simulink model "Sfun_dtc_ASR"  (Simulink 8.5)
settings: Solver=ode3  StartTime=0.0  StopTime=1  FixedStep=1e-5  RelTol=1e-3  AbsTol=1e-5
PreLoadFcn:
  | Ts=1e-5;
  | load srm64_60kw
undefined symbols (not defined in the file or in its folder): find_system
libraries: powerlib x15, simulink x1
Description:
  | Copyright 2008-2010 The MathWorks, Inc.
settings Model: Creator=MathWorks  LastModifiedBy=think0404  ExtModeAutoUpdateStatusClock=off
settings DataIOCC: SignalLoggingName=sigsOut
settings OptimizationCC: InitFltsAndDblsToZero=on
settings DebuggingCC: CheckExecutionContextPreStartOutputMsg=on  CheckExecutionContextRuntimeOutputMsg=on  SignalResolutionControl=TryResolveAllWithWarning  MultiTaskDSMMsg=warning  MultiTaskCondExecSysMsg=none  FcnCallInpInsideContextMsg=UseLocalSettings
settings HardwareCC: TargetUnknown=on

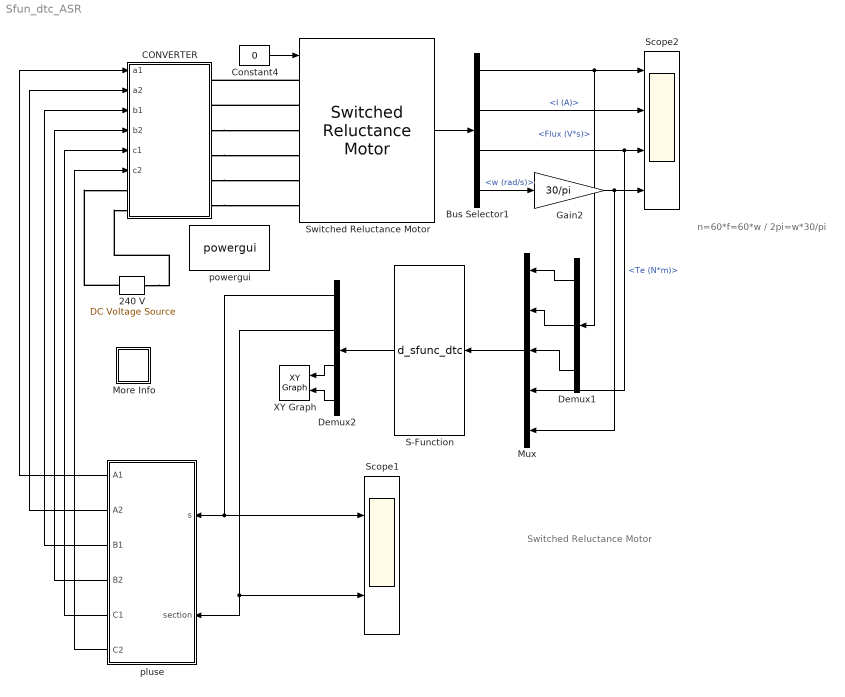
== system Sfun_dtc_ASR ==
  note: Switched Reluctance Motor
  note: n=60*f=60*w / 2pi=w*30/pi
  240 V : powerlib/Electrical Sources/DC Voltage Source  Amplitude=300  Measurements=None
  Bus Selector1 : BusSelector  OutputSignals=Flux (V*s),I (A),Te (N*m),w (rad/s)
  CONVERTER : Subsystem  LoadFcn=find_system(gcs,'FollowLinks', 'on', 'LookUnderMasks', 'all');
  Constant4 : Constant  Value=0
  Demux1 : Demux  Outputs=3
  Demux2 : Demux
  Gain2 : Gain  Gain=30/pi  SaturateOnIntegerOverflow=on  OutDataTypeStr=Inherit: Same as input  ParamDataTypeStr=Inherit: Same as input
  More Info : Subsystem
      settings: OpenFcn=showdemo(bdroot(gcb))
      mask Display: disp('?')
  Mux : Mux  Inputs=5
  S-Function : S-Function  FunctionName=d_sfunc_dtc  Parameters=0.25,3000,1e-4,1e-3,30
  Scope1 : Scope  NumInputPorts=2
      settings: TimeRange=0.1  YMin=1~1  YMax=4~6  SaveName=VI1  Decimation=10
  Scope2 : Scope  NumInputPorts=4
      settings: TimeRange=1  YMin=-0.05~-50~-200~-500  YMax=0.35~550~150~4500  SaveName=VI  Decimation=10
  Switched Reluctance Motor : powerlib/Machines/Switched Reluctance Motor  MachineType=6/4  StatorResistance=0.05  Inertia=0.05  Friction=0.02  InitialSpeed=[0,0]  TsPowergui=0  TsBlock=-1  MachineModel=Generic model  Lq=0.67e-3  Ld=23.6e-3  Lsat=0.15e-3  MaximumCurrent=450  MaximumFluxLinkage=0.486  Source=MAT-file  MagnetisationCharacteristic='srm64_60kw.mat'  RotorAngleVector=[0 10 20 30 40 45]  StatorCurrentVector=0:25:450  PlotCurves=off
  XY Graph : simulink/Sinks/XY Graph  xmin=-1  xmax=1  ymin=-1  ymax=1  st=-1
  pluse : Subsystem
  powergui : powerlib/powergui  Priority=2  SimulationMode=Discrete  SolverType=Tustin/Backward Euler (TBE)  SampleTime=1e-5  frequency=60  SPID=off  DisableSnubberDevices=off  DisableRonSwitches=off  DisableVfSwitches=off  SwTol=0  DisplayEquations=off  Interpol=off  methode=off  Ts=0  FunctionMessages=off  echomessages=off  HookPort=off  EnableUseOfTLC=off  x0status=blocks  frequencyindice=0  Pbase=100e6  ErrMax=1e-4  Iterations=50  UnitsV=kV  UnitsW=MW  buscounter=0  RestoreLinks=warning  ResistiveCurrentMeasurement=off  Frange=[0:2:500]  Ylog=off  Xlog=on  ShowGrid=off  save=off  variable=ZData  structure=0  ZoomFFT=on  StartTime=0.0  cycles=1  DisplayStyle=1  fundamental=60  FreqAxis=off  MaxFrequency=1000  frequencyindicesteady=1  RmsSteady=1  display=off
  wires:
  Constant4/1 -> Switched Reluctance Motor/1
  Switched Reluctance Motor/1 -> Bus Selector1/1
  Bus Selector1/1 -> Scope2/1, Demux1/1  "<Flux (V*s)>"
  Bus Selector1/2 -> Scope2/2  "<I (A)>"
  Bus Selector1/3 -> Scope2/3, Mux/4  "<Te (N*m)>"
  Gain2/1 -> Scope2/4, Mux/5
  Bus Selector1/4 -> Gain2/1  "<w (rad/s)>"
  pluse/1(A1) -> CONVERTER/1(a1)
  pluse/2(A2) -> CONVERTER/2(a2)
  pluse/3(B1) -> CONVERTER/3(b1)
  pluse/4(B2) -> CONVERTER/4(b2)
  pluse/5(C1) -> CONVERTER/5(c1)
  pluse/6(C2) -> CONVERTER/6(c2)
  Demux1/1 -> Mux/1
  Demux1/2 -> Mux/2
  Demux1/3 -> Mux/3
  Mux/1 -> S-Function/1
  S-Function/1 -> Demux2/1
  Demux2/1 -> pluse/1(s), Scope1/1
  Demux2/2 -> pluse/2(section), Scope1/2
  Demux2/3 -> XY Graph/1
  Demux2/4 -> XY Graph/2
  connections:
  Switched Reluctance Motor/LConn1 -- CONVERTER/RConn1
  Switched Reluctance Motor/LConn2 -- CONVERTER/RConn2
  CONVERTER/RConn3 -- Switched Reluctance Motor/LConn3
  CONVERTER/RConn4 -- Switched Reluctance Motor/LConn4
  CONVERTER/RConn5 -- Switched Reluctance Motor/LConn5
  CONVERTER/RConn6 -- Switched Reluctance Motor/LConn6
  240 V/RConn1 -- CONVERTER/LConn1
  240 V/LConn1 -- CONVERTER/LConn2

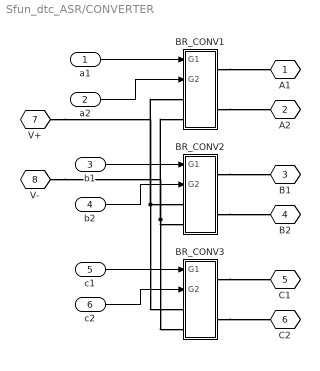
== system Sfun_dtc_ASR/CONVERTER ==
  a1 : Inport
  a2 : Inport  Port=2
  b1 : Inport  Port=3
  b2 : Inport  Port=4
  c1 : Inport  Port=5
  c2 : Inport  Port=6
  BR_CONV1 : Subsystem
  BR_CONV2 : Subsystem
  BR_CONV3 : Subsystem
  A1 : PMIOPort  Tag=PMCPort  Port=1  Side=Right
  A2 : PMIOPort  Tag=PMCPort  Port=2  Side=Right
  B1 : PMIOPort  Tag=PMCPort  Port=3  Side=Right
  B2 : PMIOPort  Tag=PMCPort  Port=4  Side=Right
  C1 : PMIOPort  Tag=PMCPort  Port=5  Side=Right
  C2 : PMIOPort  Tag=PMCPort  Port=6  Side=Right
  V+ : PMIOPort  Tag=PMCPort  Port=7  Side=Left
  V- : PMIOPort  Tag=PMCPort  Port=8  Side=Left
  wires:
  a1/1 -> BR_CONV1/1(G1)
  a2/1 -> BR_CONV1/2(G2)
  b1/1 -> BR_CONV2/1(G1)
  b2/1 -> BR_CONV2/2(G2)
  c1/1 -> BR_CONV3/1(G1)
  c2/1 -> BR_CONV3/2(G2)
  connections:
  BR_CONV3/RConn2 -- C2/RConn1
  BR_CONV3/RConn1 -- C1/RConn1
  BR_CONV2/RConn2 -- B2/RConn1
  BR_CONV2/RConn1 -- B1/RConn1
  BR_CONV1/RConn2 -- A2/RConn1
  BR_CONV1/RConn1 -- A1/RConn1
  V+/RConn1 -- BR_CONV1/LConn1 -- BR_CONV2/LConn1 -- BR_CONV3/LConn1
  V-/RConn1 -- BR_CONV1/LConn2 -- BR_CONV2/LConn2 -- BR_CONV3/LConn2

== system Sfun_dtc_ASR/More Info ==

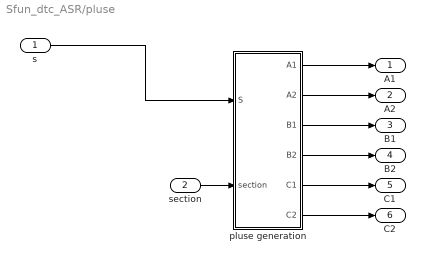
== system Sfun_dtc_ASR/pluse ==
  s : Inport
  section : Inport  Port=2
  pluse generation : Subsystem
  A1 : Outport
  A2 : Outport  Port=2
  B1 : Outport  Port=3
  B2 : Outport  Port=4
  C1 : Outport  Port=5
  C2 : Outport  Port=6
  wires:
  s/1 -> pluse generation/1(S)
  section/1 -> pluse generation/2(section)
  pluse generation/1(A1) -> A1/1
  pluse generation/2(A2) -> A2/1
  pluse generation/3(B1) -> B1/1
  pluse generation/4(B2) -> B2/1
  pluse generation/5(C1) -> C1/1
  pluse generation/6(C2) -> C2/1

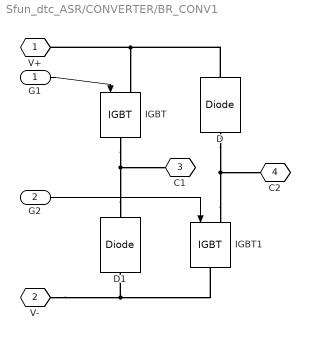
== system Sfun_dtc_ASR/CONVERTER/BR_CONV1 ==
  G1 : Inport
  G2 : Inport  Port=2
  D : powerlib/Power Electronics/Diode  Ron=1e-3  Lon=0  Vf=0.8  IC=0  UseSnubber=off  Rs=1000  Cs=inf  Measurements=off
  D1 : powerlib/Power Electronics/Diode  Ron=1e-3  Lon=0  Vf=0.8  IC=0  UseSnubber=off  Rs=1000  Cs=inf  Measurements=off
  IGBT : powerlib/Power Electronics/IGBT  Ron=1e-3  Lon=0  Vf=1  Tf=0  Tt=0  IC=0  Rs=200  Cs=0.1e-6  Measurements=off
  IGBT1 : powerlib/Power Electronics/IGBT  Ron=1e-3  Lon=0  Vf=1  Tf=0  Tt=0  IC=0  Rs=200  Cs=0.1e-6  Measurements=off
  V+ : PMIOPort  Tag=PMCPort  Port=1  Side=Left
  V- : PMIOPort  Tag=PMCPort  Port=2  Side=Left
  C1 : PMIOPort  Tag=PMCPort  Port=3  Side=Right
  C2 : PMIOPort  Tag=PMCPort  Port=4  Side=Right
  wires:
  G2/1 -> IGBT1/1
  G1/1 -> IGBT/1
  connections:
  D1/LConn1 -- V-/RConn1 -- IGBT1/RConn1
  IGBT1/LConn1 -- D/LConn1 -- C2/RConn1
  D1/RConn1 -- IGBT/RConn1 -- C1/RConn1
  D/RConn1 -- V+/RConn1 -- IGBT/LConn1

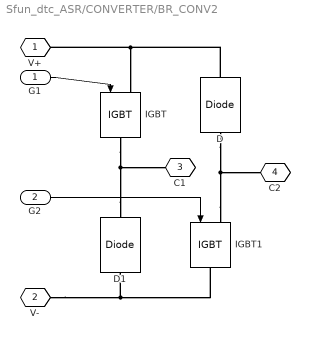
== system Sfun_dtc_ASR/CONVERTER/BR_CONV2 ==
  G1 : Inport
  G2 : Inport  Port=2
  D : powerlib/Power Electronics/Diode  Ron=1e-3  Lon=0  Vf=0.8  IC=0  UseSnubber=off  Rs=1000  Cs=inf  Measurements=off
  D1 : powerlib/Power Electronics/Diode  Ron=1e-3  Lon=0  Vf=0.8  IC=0  UseSnubber=off  Rs=1000  Cs=inf  Measurements=off
  IGBT : powerlib/Power Electronics/IGBT  Ron=1e-3  Lon=0  Vf=1  Tf=0  Tt=0  IC=0  Rs=200  Cs=0.1e-6  Measurements=off
  IGBT1 : powerlib/Power Electronics/IGBT  Ron=1e-3  Lon=0  Vf=1  Tf=0  Tt=0  IC=0  Rs=200  Cs=0.1e-6  Measurements=off
  V+ : PMIOPort  Tag=PMCPort  Port=1  Side=Left
  V- : PMIOPort  Tag=PMCPort  Port=2  Side=Left
  C1 : PMIOPort  Tag=PMCPort  Port=3  Side=Right
  C2 : PMIOPort  Tag=PMCPort  Port=4  Side=Right
  wires:
  G2/1 -> IGBT1/1
  G1/1 -> IGBT/1
  connections:
  D1/LConn1 -- V-/RConn1 -- IGBT1/RConn1
  IGBT1/LConn1 -- D/LConn1 -- C2/RConn1
  D1/RConn1 -- IGBT/RConn1 -- C1/RConn1
  D/RConn1 -- V+/RConn1 -- IGBT/LConn1

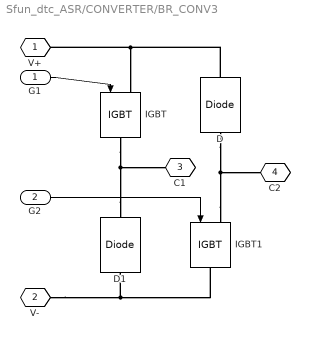
== system Sfun_dtc_ASR/CONVERTER/BR_CONV3 ==
  G1 : Inport
  G2 : Inport  Port=2
  D : powerlib/Power Electronics/Diode  Ron=1e-3  Lon=0  Vf=0.8  IC=0  UseSnubber=off  Rs=1000  Cs=inf  Measurements=off
  D1 : powerlib/Power Electronics/Diode  Ron=1e-3  Lon=0  Vf=0.8  IC=0  UseSnubber=off  Rs=1000  Cs=inf  Measurements=off
  IGBT : powerlib/Power Electronics/IGBT  Ron=1e-3  Lon=0  Vf=1  Tf=0  Tt=0  IC=0  Rs=200  Cs=0.1e-6  Measurements=off
  IGBT1 : powerlib/Power Electronics/IGBT  Ron=1e-3  Lon=0  Vf=1  Tf=0  Tt=0  IC=0  Rs=200  Cs=0.1e-6  Measurements=off
  V+ : PMIOPort  Tag=PMCPort  Port=1  Side=Left
  V- : PMIOPort  Tag=PMCPort  Port=2  Side=Left
  C1 : PMIOPort  Tag=PMCPort  Port=3  Side=Right
  C2 : PMIOPort  Tag=PMCPort  Port=4  Side=Right
  wires:
  G2/1 -> IGBT1/1
  G1/1 -> IGBT/1
  connections:
  D1/LConn1 -- V-/RConn1 -- IGBT1/RConn1
  IGBT1/LConn1 -- D/LConn1 -- C2/RConn1
  D1/RConn1 -- IGBT/RConn1 -- C1/RConn1
  D/RConn1 -- V+/RConn1 -- IGBT/LConn1

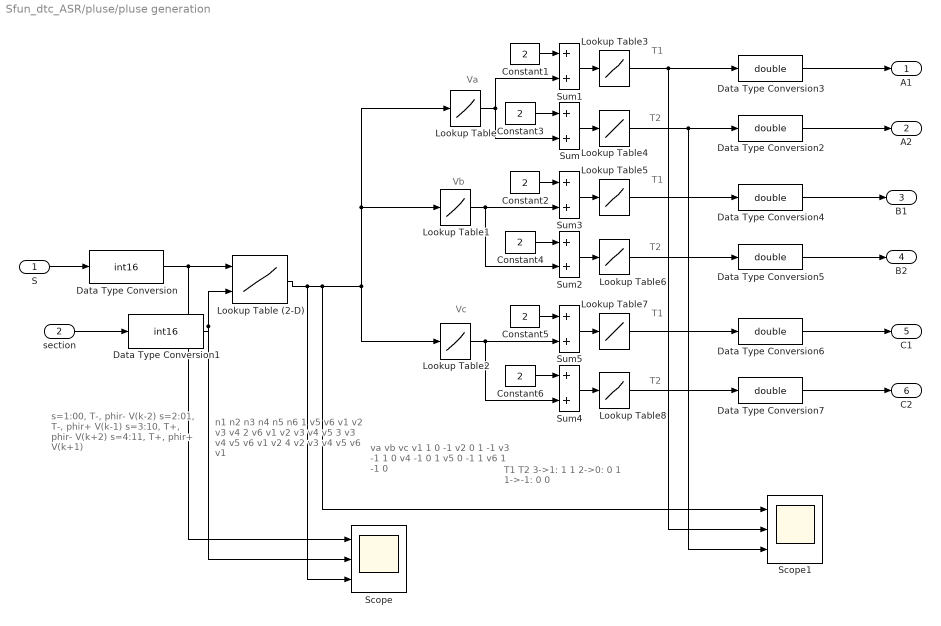
== system Sfun_dtc_ASR/pluse/pluse generation ==
  note: n1   n2  n3  n4   n5  n6
      |    1  v5   v6   v1   v2   v3   v4
      |    2  v6   v1   v2   v3   v4   v5
      |    3  v3   v4   v5   v6   v1   v2
      |   4  v2   v3   v4   v5   v6   v1
  note: s=1:00, T-,  phir-     V(k-2)
      | s=2:01, T-,  phir+     V(k-1)
      | s=3:10, T+,  phir-     V(k+2)
      | s=4:11, T+,  phir+     V(k+1)
  note: va    vb     vc
      | v1  1     0     -1
      | v2  0     1     -1
      | v3  -1     1     0
      | v4  -1     0     1
      | v5  0     -1    1
      | v6  1     -1     0
  note: T1    T2
      | 3->1:  1      1
      | 2->0:  0      1
      | 1->-1:  0      0
  note: Va
  note: Vb
  note: Vc
  note: T1
  note: T2
  note: T1
  note: T2
  note: T1
  note: T2
  S : Inport
  section : Inport  Port=2
  Constant{1..6} (6 alike) : Constant  Value=2
  Data Type Conversion : DataTypeConversion  OutDataTypeStr=int16
  Data Type Conversion1 : DataTypeConversion  OutDataTypeStr=int16
  Data Type Conversion{2..7} (6 alike) : DataTypeConversion  OutDataTypeStr=double
  Lookup Table (2-D) : Lookup2D  RowIndex=[1:4]  ColumnIndex=[1:6]  Table=[5 6 1 2 3 4;6 1 2 3 4 5;3 4 5 6 1 2;2 3 4 5 6 1]
  Lookup Table : Lookup  InputValues=[1:6]  Table=[1 0 -1 -1 0 1]
  Lookup Table1 : Lookup  InputValues=[1:6]  Table=[0 1 1 0 -1 -1]
  Lookup Table2 : Lookup  InputValues=[1:6]  Table=[-1 -1 0 1 1 0]
  Lookup Table3 : Lookup  InputValues=[1:3]  Table=[0 0 1]
  Lookup Table4 : Lookup  InputValues=[1:3]  Table=[0 1 1]
  Lookup Table5 : Lookup  InputValues=[1:3]  Table=[0 0 1]
  Lookup Table6 : Lookup  InputValues=[1:3]  Table=[0 1 1]
  Lookup Table7 : Lookup  InputValues=[1:3]  Table=[0 0 1]
  Lookup Table8 : Lookup  InputValues=[1:3]  Table=[0 1 1]
  Scope : Scope  NumInputPorts=3
      settings: YMin=4~1~1  YMax=4~6~6
  Scope1 : Scope  NumInputPorts=3
      settings: YMin=1~0~0  YMax=6~1~1
  Sum{,1..5} (6 alike) : Sum
  A1 : Outport
  A2 : Outport  Port=2
  B1 : Outport  Port=3
  B2 : Outport  Port=4
  C1 : Outport  Port=5
  C2 : Outport  Port=6
  wires:
  S/1 -> Data Type Conversion/1
  section/1 -> Data Type Conversion1/1
  Data Type Conversion/1 -> Lookup Table (2-D)/1, Scope/1
  Data Type Conversion1/1 -> Lookup Table (2-D)/2, Scope/2
  Lookup Table (2-D)/1 -> Scope/3, Lookup Table2/1, Lookup Table/1, Lookup Table1/1, Scope1/1
  Constant1/1 -> Sum1/1
  Sum1/1 -> Lookup Table3/1
  Constant3/1 -> Sum/1
  Sum/1 -> Lookup Table4/1
  Lookup Table/1 -> Sum1/2, Sum/2
  Constant2/1 -> Sum3/1
  Sum3/1 -> Lookup Table5/1
  Constant4/1 -> Sum2/1
  Sum2/1 -> Lookup Table6/1
  Lookup Table1/1 -> Sum2/2, Sum3/2
  Constant5/1 -> Sum5/1
  Sum5/1 -> Lookup Table7/1
  Constant6/1 -> Sum4/1
  Sum4/1 -> Lookup Table8/1
  Lookup Table2/1 -> Sum5/2, Sum4/2
  Lookup Table3/1 -> Data Type Conversion3/1, Scope1/2
  Lookup Table4/1 -> Data Type Conversion2/1, Scope1/3
  Lookup Table5/1 -> Data Type Conversion4/1
  Lookup Table6/1 -> Data Type Conversion5/1
  Lookup Table7/1 -> Data Type Conversion6/1
  Lookup Table8/1 -> Data Type Conversion7/1
  Data Type Conversion3/1 -> A1/1
  Data Type Conversion2/1 -> A2/1
  Data Type Conversion4/1 -> B1/1
  Data Type Conversion5/1 -> B2/1
  Data Type Conversion6/1 -> C1/1
  Data Type Conversion7/1 -> C2/1
